simulink model "Coordinated_ctrl_tuning"  (R2022a)
settings: Solver=VariableStepAuto  StartTime=0.0  StopTime=10.0  RelTol=1e-3
values from neighbouring files (symbols this model uses):
  n = sr.NumActiveJoints    [traj_tracking_6DoF.m]
  N = n + 6    [traj_tracking_6DoF.m]
undefined symbols (not defined in the file or in its folder): A, B, C, D, x0
settings Model: Creator=charl  LastModifiedBy=charl

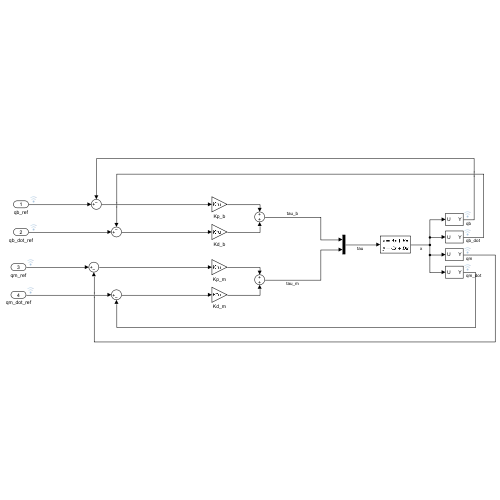
[thumbnail: Simulink's stored preview of the top-level diagram]
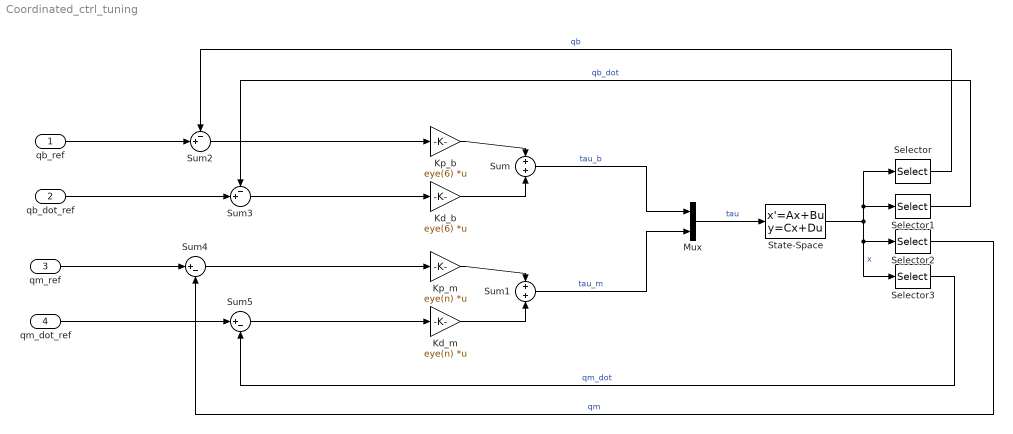
== system Coordinated_ctrl_tuning ==
  qb_ref : Inport  PortDimensions=6
  qb_dot_ref : Inport  Port=2  PortDimensions=6
  qm_ref : Inport  Port=3  PortDimensions=n
  qm_dot_ref : Inport  Port=4  PortDimensions=n
  Kd_b : Gain  Gain=eye(6)  Multiplication=Matrix(K*u)
  Kd_m : Gain  Gain=eye(n)  Multiplication=Matrix(K*u)
  Kp_b : Gain  Gain=eye(6)  Multiplication=Matrix(K*u)
  Kp_m : Gain  Gain=eye(n)  Multiplication=Matrix(K*u)
  Mux : Mux  Inputs=2
  Selector : Selector  IndexOptions=Index vector (dialog)  Indices=[1:6]  OutputSizes=1
  Selector1 : Selector  IndexOptions=Index vector (dialog)  Indices=[N+1:N+6]  OutputSizes=1
  Selector2 : Selector  IndexOptions=Index vector (dialog)  Indices=[7:6+n]  OutputSizes=1
  Selector3 : Selector  IndexOptions=Index vector (dialog)  Indices=[N+7:2*N]  OutputSizes=1
  State-Space : StateSpace  A=A  B=B  C=C  D=D  InitialCondition=x0
  Sum : Sum  Inputs=+|+
  Sum1 : Sum  Inputs=+|+
  Sum2 : Sum  Inputs=-+|
  Sum3 : Sum  Inputs=-+|
  Sum4 : Sum  Inputs=|+-
  Sum5 : Sum  Inputs=|+-
  wires:
  State-Space/1 -> Selector1/1, Selector/1, Selector3/1, Selector2/1  "x"
  Selector/1 -> Sum2/1  "qb"
  Selector1/1 -> Sum3/1  "qb_dot"
  Selector2/1 -> Sum4/2  "qm"
  Selector3/1 -> Sum5/2  "qm_dot"
  Mux/1 -> State-Space/1  "tau"
  Sum/1 -> Mux/1  "tau_b"
  Kp_b/1 -> Sum/1
  Kd_b/1 -> Sum/2
  Sum2/1 -> Kp_b/1
  Sum3/1 -> Kd_b/1
  Sum5/1 -> Kd_m/1
  Kd_m/1 -> Sum1/2
  Sum4/1 -> Kp_m/1
  Kp_m/1 -> Sum1/1
  Sum1/1 -> Mux/2  "tau_m"
  qb_ref/1 -> Sum2/2
  qb_dot_ref/1 -> Sum3/2
  qm_ref/1 -> Sum4/1
  qm_dot_ref/1 -> Sum5/1
